simulink model "Wiper_washer_final"  (R2023b)
settings: Solver=VariableStepAuto  StartTime=0.0  StopTime=100  RelTol=1e-3
libraries: spsOnDelayLib x2
settings Model: LastModifiedBy=40674
settings RTWCC: GenCodeOnly=on  GenerateReport=on  LaunchReport=on  GPUComputeCapability=5.0

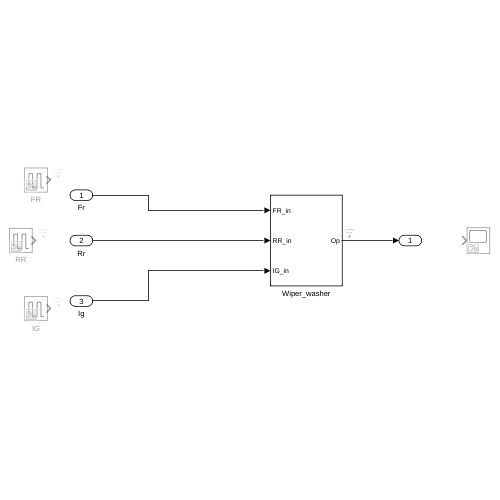
[thumbnail: Simulink's stored preview of the top-level diagram]
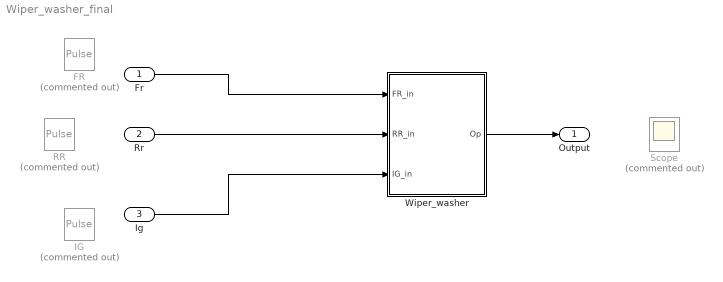
== system Wiper_washer_final ==
  Fr : Inport
  Rr : Inport  Port=2
  Ig : Inport  Port=3
  FR : DiscretePulseGenerator  Commented=on  PulseType=Time based  Amplitude=2  Period=20  PulseWidth=50  PhaseDelay=10
  IG : DiscretePulseGenerator  Commented=on  PulseType=Time based  Amplitude=4  Period=50  PulseWidth=75
  RR : DiscretePulseGenerator  Commented=on  PulseType=Time based  Period=20  PulseWidth=50  PhaseDelay=5
  Scope : Scope  Commented=on
  Wiper_washer : Subsystem
  Output : Outport
  wires:
  Wiper_washer/1(Op) -> Output/1
  Fr/1 -> Wiper_washer/1(FR_in)
  Rr/1 -> Wiper_washer/2(RR_in)
  Ig/1 -> Wiper_washer/3(IG_in)

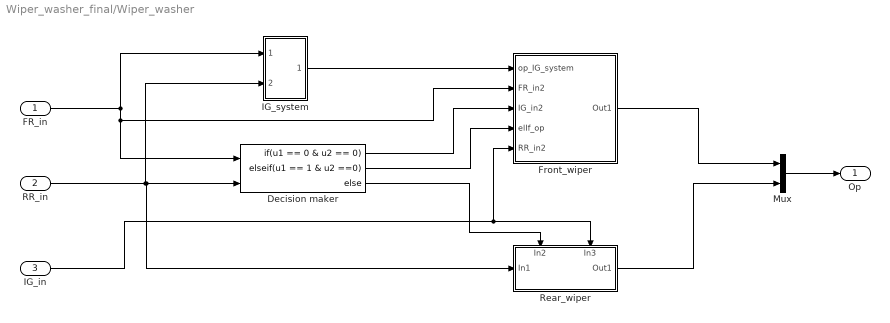
== system Wiper_washer_final/Wiper_washer ==
  FR_in : Inport
  RR_in : Inport  Port=2
  IG_in : Inport  Port=3
  Decision maker : If  NumInputs=2  IfExpression=u1 == 0 & u2 == 0  ElseIfExpressions=u1 == 1 & u2 ==0
  Front_wiper : Subsystem
  IG_system : Subsystem
  Mux : Mux  Inputs=2
  Rear_wiper : Subsystem
      settings: PortSchema="{\"entries\":[{\"content\":{\"sides\":[{\"content\":{\"connectorIds\":[\"In1\"]},\"type\":\"ConnectorPlacement.EquallySpacedRectSide\",\"uuid\":\"82858bf5-5e77-4106-a34e-58aea0a827bd\"},{\"content\":{\"connectorIds\":[\"Out1\"],\"side\":\"RIGHT\"},\"type\":\"ConnectorPlacement.EquallySpacedRectSide\",\"uuid\":\"8faf0323-7e40-42c3-9fd5-1121a901cf1d\"},{\"content\":{\"connectorIds\":[\"In2\",\"In3\"],\"side\":\"TOP\"},\"type\":\"ConnectorPlacement.EquallySpacedRectSide\",\"uuid\":\"337a5927-3ca8-4f44-a8e2-f64a97d9eb71\"}]},\"type\":\"ConnectorPlacement.EquallySpacedConnector\",\"uuid\":\"6bfac374-8f43-4f13-9a07-406bdeb0dc42\"}],\"packageUris\":[\"http://schema.mathworks.com/mf0/Connector/R2020b\"],\"version\":\"1.0\"}"
  Op : Outport
  wires:
  Decision maker/3 -> Rear_wiper/2(In2)
  RR_in/1 -> IG_system/2(In2), Rear_wiper/1(In1), Decision maker/2
  Rear_wiper/1(Out1) -> Mux/2
  FR_in/1 -> Front_wiper/2(FR_in2), Decision maker/1, IG_system/1(In1)
  IG_in/1 -> Rear_wiper/3(In3), Front_wiper/5(RR_in2)
  Mux/1 -> Op/1
  IG_system/1(Out1) -> Front_wiper/1(op_IG_system)
  Decision maker/1 -> Front_wiper/3(IG_in2)
  Decision maker/2 -> Front_wiper/4(elIf_op)
  Front_wiper/1(Out1) -> Mux/1

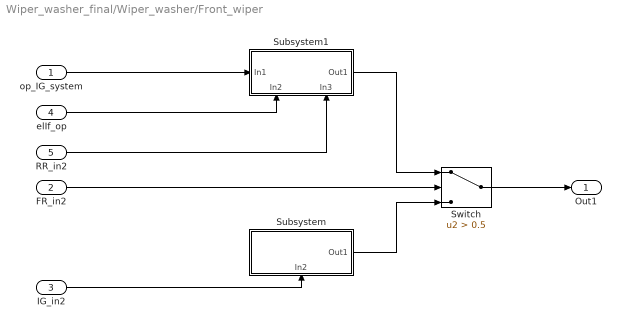
== system Wiper_washer_final/Wiper_washer/Front_wiper ==
  op_IG_system : Inport
  FR_in2 : Inport  Port=2
  IG_in2 : Inport  Port=3
  elIf_op : Inport  Port=4
  RR_in2 : Inport  Port=5
  Subsystem : Subsystem
      settings: PortSchema="{\"entries\":[{\"content\":{\"sides\":[{\"content\":{},\"type\":\"ConnectorPlacement.EquallySpacedRectSide\",\"uuid\":\"82858bf5-5e77-4106-a34e-58aea0a827bd\"},{\"content\":{\"connectorIds\":[\"Out1\"],\"side\":\"RIGHT\"},\"type\":\"ConnectorPlacement.EquallySpacedRectSide\",\"uuid\":\"8faf0323-7e40-42c3-9fd5-1121a901cf1d\"},{\"content\":{\"side\":\"TOP\"},\"type\":\"ConnectorPlacement.EquallySpacedRectSide\",\"uuid\":\"337a5927-3ca8-4f44-a8e2-f64a97d9eb71\"},{\"content\":{\"connectorIds\":[\"In1\"],\"side\":\"BOTTOM\"},\"type\":\"ConnectorPlacement.EquallySpacedRectSide\",\"uuid\":\"eeaa726f-dd0f-443f-9d1f-d047b1d9abcc\"}]},\"type\":\"ConnectorPlacement.EquallySpacedConnector\",\"uuid\":\"6bfac374-8f43-4f13-9a07-406bdeb0dc42\"}],\"packageUris\":[\"http://schema.mathworks.com/mf0/Connector/R2020b\"],\"version\":\"1.0\"}"
  Subsystem1 : Subsystem
      settings: PortSchema="{\"entries\":[{\"content\":{\"sides\":[{\"content\":{\"connectorIds\":[\"In1\"]},\"type\":\"ConnectorPlacement.EquallySpacedRectSide\",\"uuid\":\"82858bf5-5e77-4106-a34e-58aea0a827bd\"},{\"content\":{\"connectorIds\":[\"Out1\"],\"side\":\"RIGHT\"},\"type\":\"ConnectorPlacement.EquallySpacedRectSide\",\"uuid\":\"8faf0323-7e40-42c3-9fd5-1121a901cf1d\"},{\"content\":{\"side\":\"TOP\"},\"type\":\"ConnectorPlacement.EquallySpacedRectSide\",\"uuid\":\"337a5927-3ca8-4f44-a8e2-f64a97d9eb71\"},{\"content\":{\"connectorIds\":[\"In2\",\"In3\"],\"side\":\"BOTTOM\"},\"type\":\"ConnectorPlacement.EquallySpacedRectSide\",\"uuid\":\"9fdd98a8-874b-4aac-81df-cd8539f5d395\"}]},\"type\":\"ConnectorPlacement.EquallySpacedConnector\",\"uuid\":\"6bfac374-8f43-4f13-9a07-406bdeb0dc42\"}],\"packageUris\":[\"http://schema.mathworks.com/mf0/Connector/R2020b\"],\"version\":\"1.0\"}"
  Switch : Switch  Criteria=u2 > Threshold  Threshold=0.5  SaturateOnIntegerOverflow=off  InputSameDT=off
  Out1 : Outport
  wires:
  FR_in2/1 -> Switch/2
  Subsystem/1(Out1) -> Switch/3
  Subsystem1/1(Out1) -> Switch/1
  Switch/1 -> Out1/1
  RR_in2/1 -> Subsystem1/3(In3)
  op_IG_system/1 -> Subsystem1/1(In1)
  elIf_op/1 -> Subsystem1/2(In2)
  IG_in2/1 -> Subsystem/1(In2)

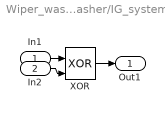
== system Wiper_washer_final/Wiper_washer/IG_system ==
  In1 : Inport
  In2 : Inport  Port=2
  XOR : Logic  Operator=XOR  IconShape=distinctive  AllPortsSameDT=off  OutDataTypeStr=boolean
  Out1 : Outport
  wires:
  In1/1 -> XOR/1
  XOR/1 -> Out1/1
  In2/1 -> XOR/2

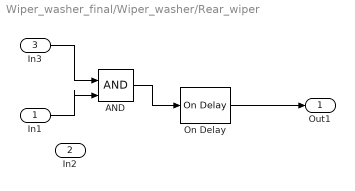
== system Wiper_washer_final/Wiper_washer/Rear_wiper ==
  In1 : Inport
  In2 : Inport  Port=2
  In3 : Inport  Port=3
  AND : Logic  IconShape=distinctive  AllPortsSameDT=off  OutDataTypeStr=boolean
  On Delay : spsOnDelayLib/On Delay  DelayType=On delay  delay=1  ic=0  Ts=0
  Out1 : Outport
  wires:
  In1/1 -> AND/2
  On Delay/1 -> Out1/1
  AND/1 -> On Delay/1
  In3/1 -> AND/1

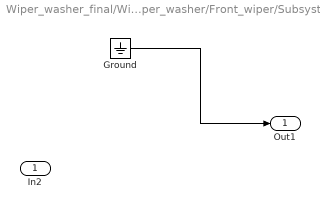
== system Wiper_washer_final/Wiper_washer/Front_wiper/Subsystem ==
  In2 : Inport
  Ground : Ground
  Out1 : Outport
  wires:
  Ground/1 -> Out1/1

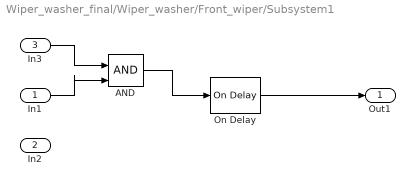
== system Wiper_washer_final/Wiper_washer/Front_wiper/Subsystem1 ==
  In1 : Inport
  In2 : Inport  Port=2
  In3 : Inport  Port=3
  AND : Logic  IconShape=distinctive  AllPortsSameDT=off  OutDataTypeStr=boolean
  On Delay : spsOnDelayLib/On Delay  DelayType=On delay  delay=1  ic=0  Ts=0
  Out1 : Outport
  wires:
  In1/1 -> AND/2
  On Delay/1 -> Out1/1
  In3/1 -> AND/1
  AND/1 -> On Delay/1
